simulink model "Iek2"  (Simulink 5.0)
settings: Solver=FixedStepDiscrete  StartTime=0.0  StopTime=10000000.0  RelTol=1e-3
libraries: simulink x2
settings Model: Creator=scaife  LastModifiedBy=scaife  ExtModeAutoUpdateStatusClock=off

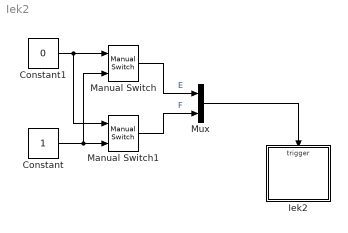
== system Iek2 ==
  Constant : Constant
  Constant1 : Constant  Value=0
  Iek2 : Stateflow chart
  Manual Switch : simulink/Signal Routing/Manual Switch  sw=1  action=0
  Manual Switch1 : simulink/Signal Routing/Manual Switch  sw=1  action=0
  Mux : Mux  Inputs=2
  wires:
  Constant1/1 -> Manual Switch/1, Manual Switch1/1
  Constant/1 -> Manual Switch1/2, Manual Switch/2
  Manual Switch1/1 -> Mux/2  "F"
  Manual Switch/1 -> Mux/1  "E"
  Mux/1 -> Iek2/Trigger

== stateflow chart Iek2 ==
  state T1 [parallel]
    state B
    state A
    (default) -> A
    A -> B : E{x++}
    B -> A : E{x++}
  state T2 [parallel]
    state C/
      en: y++
    state D/
      en: y++
    (default) -> C
    D -> C : F
    C -> D : F
  state T3 [parallel]
    state a
    state c
    state b
    state d
    (default) -> a
    a -> c : change(x)
    c -> d : change(x)
    d -> b : change(y)
    b -> a : change(y)
    c -> b : change(y)
    b -> c : change(x)
  data: x local int8; y local int8
  events: E input EITHER_EDGE_EVENT; F input EITHER_EDGE_EVENT
